simulink model "final_sim"  (R2025a)
settings: Solver=ode45  StartTime=0.0  StopTime=15  FixedStep=T  MaxStep=0.01  RelTol=1e-12  AbsTol=1e-12  EnableMultiTasking=on
values from neighbouring files (symbols this model uses):
  beam_T = 0.36    [final_sim_params.mat]
  gear_T = 0.004    [final_sim_params.mat]
  k_1 = -3.11083    [final_sim_params.mat]
  k_2 = 0.06091    [WORKING_BACKUP.mat]    (also in final_sim_params.mat; iop_control_design_integrator.m)
  k_3 = -4.25    [WORKING_BACKUP.mat]    (also in final_sim_params.mat; iop_control_design_integrator.m = -4.0162)
  tau = 0.04328    [final_sim_params.mat]
libraries: cstblocks x2
settings Model: Creator=cnielsen  LastModifiedBy=lucs1
settings SolverCC: AutoScaleAbsTol=off  AlgebraicLoopSolver=TrustRegion
settings DataIOCC: SaveFormat=Array  SignalLoggingSaveFormat=ModelDataLogs  SaveOutput=off  SaveTime=off  ReturnWorkspaceOutputs=off  Refine=5
settings OptimizationCC: ExpressionDepthLimit=2147483647.0  LifeSpan=inf
settings DebuggingCC: UnderspecifiedInitializationDetection=Classic  MergeDetectMultiDrivingBlocksExec=none  SolverPrmCheckMsg=warning  FcnCallInpInsideContextMsg=warning  UnconnectedInputMsg=warning  UnconnectedOutputMsg=warning  UnconnectedLineMsg=warning  StateNameClashWarn=warning  SFUnexpectedBacktrackingDiag=warning  SFNoUnconditionalDefaultTransitionDiag=warning  SFExecutionAtInitializationDiag=none  ArithmeticOperatorsInVariantConditions=warning
settings HardwareCC: ProdBitPerPointer=32.0  ProdBitPerSizeT=32.0  ProdBitPerPtrDiffT=32.0  ProdLargestAtomicFloat=None  ProdIntDivRoundTo=Undefined  ProdEndianess=Unspecified  ProdWordSize=32.0  ProdHWDeviceType=32-bit Generic
settings ModelReferenceCC: PropagateSignalLabelsOutOfModel=off
settings SFSimCC: SimUseLocalCustomCode=off  CustomCodeUndefinedFunction=UseInterfaceOnly
settings RTWCC: RTWUseLocalCustomCode=off  GPUComputeCapability=3.5
settings CodeAppCC: StateflowObjectComments=on
settings GRTTargetCC: TargetLangStandard=C89/C90 (ANSI)  CombineOutputUpdateFcns=off  GRTInterface=on
settings ConfigComp: CovMetricSettings=dw  CovSaveCumulativeToWorkspaceVar=on  CovSaveSingleToWorkspaceVar=on  CovExternalEMLEnable=off

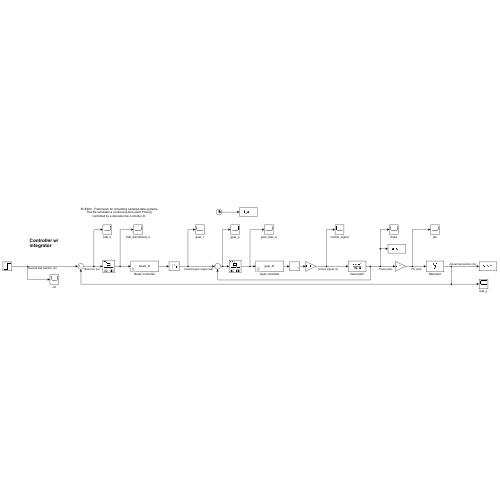
[thumbnail: Simulink's stored preview of the top-level diagram]
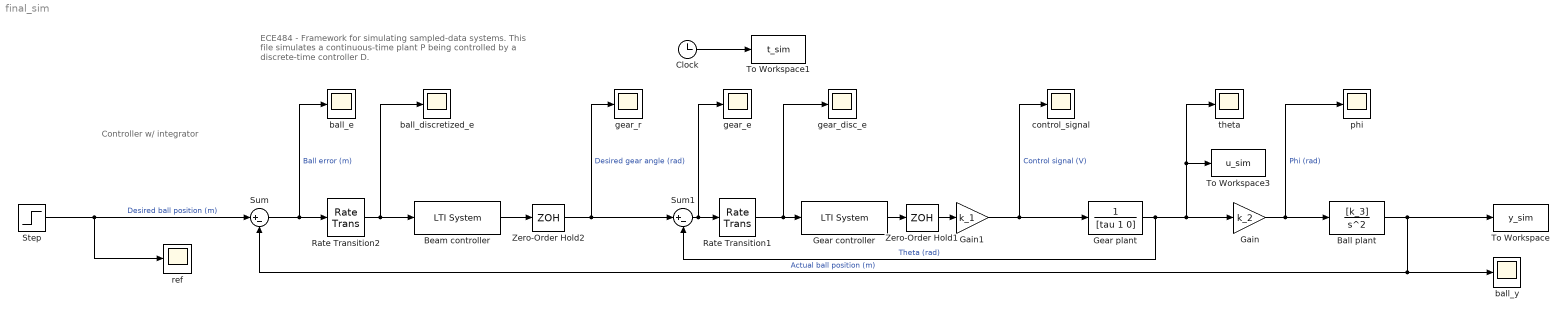
== system final_sim ==
  note: ECE484 - Framework for simulating sampled-data systems.
      | This file simulates a continuous-time plant P being
      | controlled by a discrete-time controller D.
  note: Controller w/ integrator
  Ball plant : TransferFcn  Numerator=[k_3]  Denominator=[1 0 0]
  Beam controller : cstblocks/LTI System  sys=beam_D  IC=[]  PadeOrder=0
  Clock : Clock
  Gain : Gain  Gain=k_2
  Gain1 : Gain  Gain=k_1
  Gear controller : cstblocks/LTI System  sys=gear_D  IC=[]  PadeOrder=0
  Gear plant : TransferFcn  Denominator=[tau 1 0]
  Rate Transition1 : RateTransition  OutPortSampleTime=gear_T
  Rate Transition2 : RateTransition  OutPortSampleTime=gear_T
  Step : Step  Time=0  Before=0.1  After=0.25  SampleTime=beam_T
  Sum : Sum  Inputs=|+-
  Sum1 : Sum  Inputs=|+-
  To Workspace : ToWorkspace  VariableName=y_sim  SampleTime=-1
  To Workspace1 : ToWorkspace  VariableName=t_sim  SampleTime=-1
  To Workspace3 : ToWorkspace  VariableName=u_sim  SampleTime=-1
  Zero-Order Hold1 : ZeroOrderHold  SampleTime=gear_T
  Zero-Order Hold2 : ZeroOrderHold  SampleTime=beam_T
  ball_discretized_e : Scope
      settings: ActiveDisplayYMinimum=-0.17771929278325427  ActiveDisplayYMaximum=0.297524365864806
  ball_e : Scope
      settings: ActiveDisplayYMinimum=-0.1508192120751386  ActiveDisplayYMaximum=0.29453546800834873
  ball_y : Scope
      settings: ActiveDisplayYMinimum=-0.0679732294513794  ActiveDisplayYMaximum=0.41033394929584704  DataLoggingVariableName=ScopeData2
  control_signal : Scope
      settings: ActiveDisplayYMinimum=-18.52737587654768  ActiveDisplayYMaximum=22.704310447758754  DataLoggingVariableName=ScopeData8
  gear_disc_e : Scope
      settings: ActiveDisplayYMinimum=-15.91123  ActiveDisplayYMaximum=20.79205  DataLoggingVariableName=ScopeData4
  gear_e : Scope
      settings: ActiveDisplayYMinimum=-1.4888648419330779  ActiveDisplayYMaximum=1.9001671096698076  DataLoggingVariableName=ScopeData7
  gear_r : Scope
      settings: ActiveDisplayYMinimum=-1.4336056813929809  ActiveDisplayYMaximum=1.402834664808936
  phi : Scope
      settings: ActiveDisplayYMinimum=-0.09609099624241621  ActiveDisplayYMaximum=0.077988379870732927  DataLoggingVariableName=ScopeData6
  ref : Scope
      settings: ActiveDisplayYMinimum=0.15  ActiveDisplayYMaximum=0.35  DataLoggingVariableName=ScopeData3
  theta : Scope
      settings: ActiveDisplayYMinimum=-1.5940800424194972  ActiveDisplayYMaximum=1.4287990829574659  DataLoggingVariableName=ScopeData5
  wires:
  Clock/1 -> To Workspace1/1
  Step/1 -> ref/1, Sum/1  "Desired ball position (m)"
  Sum/1 -> Rate Transition2/1, ball_e/1  "Ball error (m)"
  Rate Transition2/1 -> Beam controller/1, ball_discretized_e/1
  Gear controller/1 -> Zero-Order Hold1/1
  Rate Transition1/1 -> gear_disc_e/1, Gear controller/1
  Zero-Order Hold2/1 -> Sum1/1, gear_r/1  "Desired gear angle (rad)"
  Beam controller/1 -> Zero-Order Hold2/1
  Ball plant/1 -> ball_y/1, Sum/2, To Workspace/1  "Actual ball position (m)"
  Sum1/1 -> gear_e/1, Rate Transition1/1
  Gear plant/1 -> Gain/1, To Workspace3/1, theta/1, Sum1/2  "Theta (rad)"
  Zero-Order Hold1/1 -> Gain1/1
  Gain1/1 -> Gear plant/1, control_signal/1  "Control signal (V)"
  Gain/1 -> Ball plant/1, phi/1  "Phi (rad)"
